simulink model "powerfrompropagatorLoLaSatB"  (R2023b)
settings: Solver=FixedStepAuto  StartTime=0.0  StopTime=t_sim  FixedStep=TimeStep  RelTol=1e-3
undefined symbols (not defined in the file or in its folder): angle_roll, att, date, juliandate, LLSataero, MODE, Psa_X, Psa_Y, PsaX, PsaY
libraries: dspmathops x17, vrlib x12, aerolibutil x11, sharedtransform x9, sharedutil x4
(part 2 of 2)

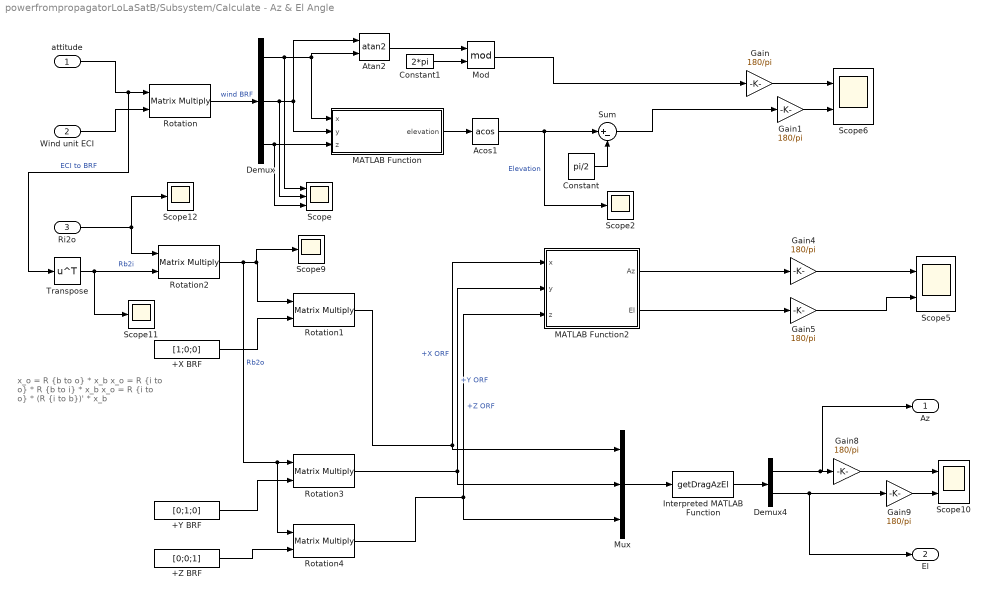
== system powerfrompropagatorLoLaSatB/Subsystem/Calculate - Az & El Angle ==
  note: x_o = R {b to o} * x_b
      | x_o = R {i to o} * R {b to i} * x_b
      | x_o = R {i to o} * (R {i to b})' * x_b
  attitude : Inport
  Wind unit ECI : Inport  Port=2
  Ri2o : Inport  Port=3
  +X BRF : Constant  Value=[1;0;0]
  +Y BRF : Constant  Value=[0;1;0]
  +Z BRF : Constant  Value=[0;0;1]
  Acos1 : Trigonometry  Operator=acos
  Atan2 : Trigonometry  Operator=atan2
  Constant : Constant  Value=pi/2
  Constant1 : Constant  Value=2*pi
  Demux : Demux  Outputs=3
  Demux4 : Demux  Outputs=2
  Gain{,1,4..5,8..9} (6 alike) : Gain  Gain=180/pi
  Interpreted MATLAB Function : MATLABFcn  MATLABFcn=getDragAzEl
  MATLAB Function : MATLAB Function  TreatAsAtomicUnit=on
  MATLAB Function2 : MATLAB Function  TreatAsAtomicUnit=on
  Mod : Math  Operator=mod  OutMin=[0]  OutMax=[2*pi]
  Mux : Mux  Inputs=3
  Rotation{,1..4} (5 alike) : Product  Multiplication=Matrix(*)  RndMeth=Zero
  Scope : Scope  NumInputPorts=3
  Scope10 : Scope  NumInputPorts=2
  Scope{2,9,11..12} (4 alike) : Scope
  Scope5 : Scope  NumInputPorts=2
  Scope6 : Scope  NumInputPorts=2
  Sum : Sum  Inputs=|+-
  Transpose : Math  Operator=transpose
  Az : Outport
  El : Outport  Port=2
  wires:
  attitude/1 -> Transpose/1, Rotation/1  "ECI to BRF"
  Wind unit ECI/1 -> Rotation/2
  Mod/1 -> Gain/1
  Constant1/1 -> Mod/2
  Atan2/1 -> Mod/1
  MATLAB Function/1(elevation) -> Acos1/1
  Sum/1 -> Gain1/1
  Acos1/1 -> Scope2/1, Sum/1  "Elevation"
  Demux/3 -> Scope/3, MATLAB Function/3(z)
  Rotation/1 -> Demux/1  "wind BRF"
  Demux/2 -> Scope/2, MATLAB Function/2(y), Atan2/1
  Constant/1 -> Sum/2
  Demux/1 -> Scope/1, Atan2/2, MATLAB Function/1(x)
  Gain/1 -> Scope6/1
  Gain1/1 -> Scope6/2
  Ri2o/1 -> Rotation2/1, Scope12/1
  +X BRF/1 -> Rotation1/2
  Rotation1/1 -> Mux/1, MATLAB Function2/1(x)  "+X ORF"
  Transpose/1 -> Scope11/1, Rotation2/2  "Rb2i"
  Rotation2/1 -> Rotation4/1, Rotation3/1, Scope9/1, Rotation1/1  "Rb2o"
  +Y BRF/1 -> Rotation3/2
  Rotation3/1 -> Mux/2, MATLAB Function2/2(y)  "+Y ORF"
  +Z BRF/1 -> Rotation4/2
  MATLAB Function2/2(El) -> Gain5/1
  Gain4/1 -> Scope5/1
  Gain5/1 -> Scope5/2
  MATLAB Function2/1(Az) -> Gain4/1
  Rotation4/1 -> Mux/3, MATLAB Function2/3(z)  "+Z ORF"
  Mux/1 -> Interpreted MATLAB Function/1
  Interpreted MATLAB Function/1 -> Demux4/1
  Gain9/1 -> Scope10/2
  Demux4/2 -> El/1, Gain9/1
  Demux4/1 -> Az/1, Gain8/1
  Gain8/1 -> Scope10/1

== matlab function powerfrompropagatorLoLaSatB/Subsystem/Calculate - Az & El Angle/MATLAB Function2 ==
  data: x input; Az output; y input; z input; El output
function [Az,El] = fcn(x,y,z)
%first normalize vectors: xorf, yorf, zorf
x=x/norm(x);
y=y/norm(y);
z=z/norm(z);

%2. calculate azimuth angle A, it can be found by considering the
%projection of xorf onto the xy-plane, A = arctan(xorf_y / xorf_x), where
%xorf_y and x_orf,x are the y and x compoennts of xorf respectively
if x(1)<0.1
    Az=atan2(y(2),y(1));
    if Az<0
        Az=Az+2*pi;
    end
    % Rz = [cos(Az) -sin(Az) 0;
    %       sin(Az) cos(Az) 0;
    %       0 0 1];
else
    Az=atan2(x(2),x(1));
    if Az<0
        Az = Az + 2*pi;
    end
end


%3. Rotate the vectors by Az on the Z axis 
Rz = [cos(Az)   -sin(Az)    0;
    sin(Az)     cos(Az)     0;
    0           0           1];
xrot=Rz*[1;0;0];
xrot=xrot/(norm(xrot));
%yrot=Rz*y;
%zrot=Rz*[0;0;1];


%4. Calculate the Elevation angle E:
%it is the angle that rotates the rotated vectors by a rotation on the Y
%axis, this angle can be found by considering the angle between xrot and
%xorf. El = acos (xrot*xorf / norm(xrot)*norm(xorf))
product=dot(xrot,x);
    if product<0
        El=-acos(product);
    else
        El=acos(product);
    end
% El = acos(dot(xrot,x));
%%El=pi/2-acos(dot(zrot,z));
    % if(z(3))<0
    %     El = -acos(z(3));
    % else
    %     El = acos(z(3));
    % end
end

== matlab function powerfrompropagatorLoLaSatB/Subsystem/Calculate - Az & El Angle/MATLAB Function ==
  data: x input; elevation output; y input; z input
function elevation = fcn(x,y,z)

elevation = z/sqrt(x^2 + y^2 + z^2);
